simulink model "TST_ExtDem_SelectParameter"  (R2016b)
settings: Solver=FixedStepDiscrete  StartTime=0.0  StopTime=simTime  FixedStep=sampleTime  RelTol=1e-3
values from neighbouring files (symbols this model uses):
  testCase = 1    [initTST_ExtDem_SelectParameter_001.m]
libraries: simulink x34, UnitTest_Lib x32
(part 1 of 2)
settings Model: Creator=dulinggang  LastModifiedBy=dulinggang
settings DebuggingCC: SignalRangeChecking=error

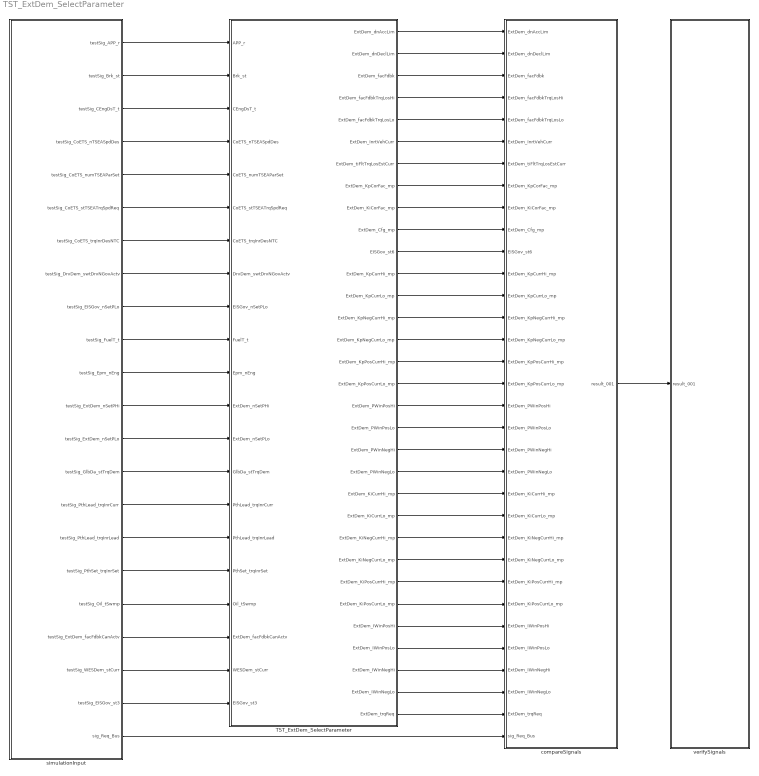
== system TST_ExtDem_SelectParameter ==
  TST_ExtDem_SelectParameter : Subsystem
  compareSignals : Subsystem
  simulationInput : Subsystem
  verifySignals : Subsystem
  wires:
  simulationInput/1(testSig_APP_r) -> TST_ExtDem_SelectParameter/1(APP_r)
  simulationInput/2(testSig_Brk_st) -> TST_ExtDem_SelectParameter/2(Brk_st)
  simulationInput/3(testSig_CEngDsT_t) -> TST_ExtDem_SelectParameter/3(CEngDsT_t)
  simulationInput/4(testSig_CoETS_nTSEASpdDes) -> TST_ExtDem_SelectParameter/4(CoETS_nTSEASpdDes)
  simulationInput/5(testSig_CoETS_numTSEAParSet) -> TST_ExtDem_SelectParameter/5(CoETS_numTSEAParSet)
  simulationInput/6(testSig_CoETS_stTSEATrqSpdReq) -> TST_ExtDem_SelectParameter/6(CoETS_stTSEATrqSpdReq)
  simulationInput/7(testSig_CoETS_trqInrDesNTC) -> TST_ExtDem_SelectParameter/7(CoETS_trqInrDesNTC)
  simulationInput/8(testSig_DrvDem_swtDrvNGovActv) -> TST_ExtDem_SelectParameter/8(DrvDem_swtDrvNGovActv)
  simulationInput/9(testSig_EISGov_nSetPLo) -> TST_ExtDem_SelectParameter/9(EISGov_nSetPLo)
  simulationInput/10(testSig_FuelT_t) -> TST_ExtDem_SelectParameter/10(FuelT_t)
  simulationInput/11(testSig_Epm_nEng) -> TST_ExtDem_SelectParameter/11(Epm_nEng)
  simulationInput/12(testSig_ExtDem_nSetPHi) -> TST_ExtDem_SelectParameter/12(ExtDem_nSetPHi)
  simulationInput/13(testSig_ExtDem_nSetPLo) -> TST_ExtDem_SelectParameter/13(ExtDem_nSetPLo)
  simulationInput/14(testSig_GlbDa_stTrqDem) -> TST_ExtDem_SelectParameter/14(GlbDa_stTrqDem)
  simulationInput/15(testSig_PthLead_trqInrCurr) -> TST_ExtDem_SelectParameter/15(PthLead_trqInrCurr)
  simulationInput/16(testSig_PthLead_trqInrLead) -> TST_ExtDem_SelectParameter/16(PthLead_trqInrLead)
  simulationInput/17(testSig_PthSet_trqInrSet) -> TST_ExtDem_SelectParameter/17(PthSet_trqInrSet)
  simulationInput/18(testSig_Oil_tSwmp) -> TST_ExtDem_SelectParameter/18(Oil_tSwmp)
  simulationInput/19(testSig_ExtDem_facFdbkCanActv) -> TST_ExtDem_SelectParameter/19(ExtDem_facFdbkCanActv)
  simulationInput/20(testSig_WESDem_stCurr) -> TST_ExtDem_SelectParameter/20(WESDem_stCurr)
  simulationInput/21(testSig_EISGov_st3) -> TST_ExtDem_SelectParameter/21(EISGov_st3)
  TST_ExtDem_SelectParameter/1(ExtDem_dnAccLim) -> compareSignals/1(ExtDem_dnAccLim)
  TST_ExtDem_SelectParameter/2(ExtDem_dnDeclLim) -> compareSignals/2(ExtDem_dnDeclLim)
  TST_ExtDem_SelectParameter/3(ExtDem_facFdbk) -> compareSignals/3(ExtDem_facFdbk)
  TST_ExtDem_SelectParameter/4(ExtDem_facFdbkTrqLosHi) -> compareSignals/4(ExtDem_facFdbkTrqLosHi)
  TST_ExtDem_SelectParameter/5(ExtDem_facFdbkTrqLosLo) -> compareSignals/5(ExtDem_facFdbkTrqLosLo)
  TST_ExtDem_SelectParameter/6(ExtDem_InrtVehCurr) -> compareSignals/6(ExtDem_InrtVehCurr)
  TST_ExtDem_SelectParameter/7(ExtDem_tiFltTrqLosEstCurr) -> compareSignals/7(ExtDem_tiFltTrqLosEstCurr)
  TST_ExtDem_SelectParameter/8(ExtDem_KpCorFac_mp) -> compareSignals/8(ExtDem_KpCorFac_mp)
  TST_ExtDem_SelectParameter/9(ExtDem_KiCorFac_mp) -> compareSignals/9(ExtDem_KiCorFac_mp)
  TST_ExtDem_SelectParameter/10(ExtDem_Cfg_mp) -> compareSignals/10(ExtDem_Cfg_mp)
  TST_ExtDem_SelectParameter/11(EISGov_st6) -> compareSignals/11(EISGov_st6)
  TST_ExtDem_SelectParameter/12(ExtDem_KpCurrHi_mp) -> compareSignals/12(ExtDem_KpCurrHi_mp)
  TST_ExtDem_SelectParameter/13(ExtDem_KpCurrLo_mp) -> compareSignals/13(ExtDem_KpCurrLo_mp)
  TST_ExtDem_SelectParameter/14(ExtDem_KpNegCurrHi_mp) -> compareSignals/14(ExtDem_KpNegCurrHi_mp)
  TST_ExtDem_SelectParameter/15(ExtDem_KpNegCurrLo_mp) -> compareSignals/15(ExtDem_KpNegCurrLo_mp)
  TST_ExtDem_SelectParameter/16(ExtDem_KpPosCurrHi_mp) -> compareSignals/16(ExtDem_KpPosCurrHi_mp)
  TST_ExtDem_SelectParameter/17(ExtDem_KpPosCurrLo_mp) -> compareSignals/17(ExtDem_KpPosCurrLo_mp)
  TST_ExtDem_SelectParameter/18(ExtDem_PWinPosHi) -> compareSignals/18(ExtDem_PWinPosHi)
  TST_ExtDem_SelectParameter/19(ExtDem_PWinPosLo) -> compareSignals/19(ExtDem_PWinPosLo)
  TST_ExtDem_SelectParameter/20(ExtDem_PWinNegHi) -> compareSignals/20(ExtDem_PWinNegHi)
  TST_ExtDem_SelectParameter/21(ExtDem_PWinNegLo) -> compareSignals/21(ExtDem_PWinNegLo)
  TST_ExtDem_SelectParameter/22(ExtDem_KiCurrHi_mp) -> compareSignals/22(ExtDem_KiCurrHi_mp)
  TST_ExtDem_SelectParameter/23(ExtDem_KiCurrLo_mp) -> compareSignals/23(ExtDem_KiCurrLo_mp)
  TST_ExtDem_SelectParameter/24(ExtDem_KiNegCurrHi_mp) -> compareSignals/24(ExtDem_KiNegCurrHi_mp)
  TST_ExtDem_SelectParameter/25(ExtDem_KiNegCurrLo_mp) -> compareSignals/25(ExtDem_KiNegCurrLo_mp)
  TST_ExtDem_SelectParameter/26(ExtDem_KiPosCurrHi_mp) -> compareSignals/26(ExtDem_KiPosCurrHi_mp)
  TST_ExtDem_SelectParameter/27(ExtDem_KiPosCurrLo_mp) -> compareSignals/27(ExtDem_KiPosCurrLo_mp)
  TST_ExtDem_SelectParameter/28(ExtDem_IWinPosHi) -> compareSignals/28(ExtDem_IWinPosHi)
  TST_ExtDem_SelectParameter/29(ExtDem_IWinPosLo) -> compareSignals/29(ExtDem_IWinPosLo)
  TST_ExtDem_SelectParameter/30(ExtDem_IWinNegHi) -> compareSignals/30(ExtDem_IWinNegHi)
  TST_ExtDem_SelectParameter/31(ExtDem_IWinNegLo) -> compareSignals/31(ExtDem_IWinNegLo)
  TST_ExtDem_SelectParameter/32(ExtDem_trqReq) -> compareSignals/32(ExtDem_trqReq)
  simulationInput/22(sig_Req_Bus) -> compareSignals/33(sig_Req_Bus)
  compareSignals/1(result_001) -> verifySignals/1(result_001)

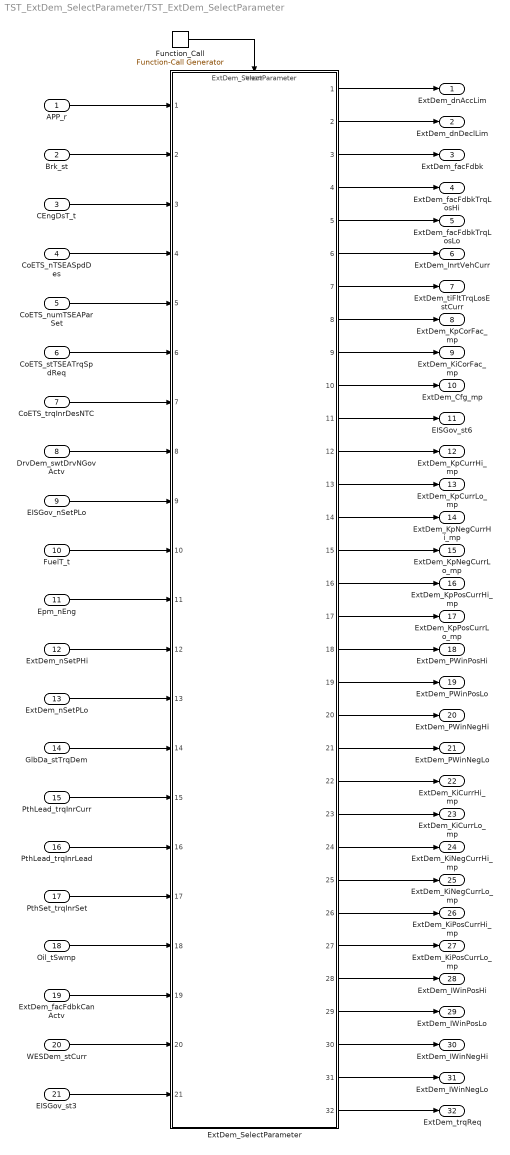
== system TST_ExtDem_SelectParameter/TST_ExtDem_SelectParameter ==
  APP_r : Inport
  Brk_st : Inport  Port=2
  CEngDsT_t : Inport  Port=3
  CoETS_nTSEASpdDes : Inport  Port=4
  CoETS_numTSEAParSet : Inport  Port=5
  CoETS_stTSEATrqSpdReq : Inport  Port=6
  CoETS_trqInrDesNTC : Inport  Port=7
  DrvDem_swtDrvNGovActv : Inport  Port=8
  EISGov_nSetPLo : Inport  Port=9
  FuelT_t : Inport  Port=10
  Epm_nEng : Inport  Port=11
  ExtDem_nSetPHi : Inport  Port=12
  ExtDem_nSetPLo : Inport  Port=13
  GlbDa_stTrqDem : Inport  Port=14
  PthLead_trqInrCurr : Inport  Port=15
  PthLead_trqInrLead : Inport  Port=16
  PthSet_trqInrSet : Inport  Port=17
  Oil_tSwmp : Inport  Port=18
  ExtDem_facFdbkCanActv : Inport  Port=19
  WESDem_stCurr : Inport  Port=20
  EISGov_st3 : Inport  Port=21
  ExtDem_SelectParameter : ModelReference  ModelNameDialog=ExtDem_SelectParameter  SimulationMode=Normal  ModelReferenceVersion=1.171  TriggerPortName=function  TriggerPortTriggerType=function-call  TriggerPortStatesWhenEnabling=held
  Function_Call : simulink/Ports & Subsystems/Function-Call Generator  sample_time=sampleTime  numberOfIterations=1
  ExtDem_dnAccLim : Outport
  ExtDem_dnDeclLim : Outport  Port=2
  ExtDem_facFdbk : Outport  Port=3
  ExtDem_facFdbkTrqLosHi : Outport  Port=4
  ExtDem_facFdbkTrqLosLo : Outport  Port=5
  ExtDem_InrtVehCurr : Outport  Port=6
  ExtDem_tiFltTrqLosEstCurr : Outport  Port=7
  ExtDem_KpCorFac_mp : Outport  Port=8
  ExtDem_KiCorFac_mp : Outport  Port=9
  ExtDem_Cfg_mp : Outport  Port=10
  EISGov_st6 : Outport  Port=11
  ExtDem_KpCurrHi_mp : Outport  Port=12
  ExtDem_KpCurrLo_mp : Outport  Port=13
  ExtDem_KpNegCurrHi_mp : Outport  Port=14
  ExtDem_KpNegCurrLo_mp : Outport  Port=15
  ExtDem_KpPosCurrHi_mp : Outport  Port=16
  ExtDem_KpPosCurrLo_mp : Outport  Port=17
  ExtDem_PWinPosHi : Outport  Port=18
  ExtDem_PWinPosLo : Outport  Port=19
  ExtDem_PWinNegHi : Outport  Port=20
  ExtDem_PWinNegLo : Outport  Port=21
  ExtDem_KiCurrHi_mp : Outport  Port=22
  ExtDem_KiCurrLo_mp : Outport  Port=23
  ExtDem_KiNegCurrHi_mp : Outport  Port=24
  ExtDem_KiNegCurrLo_mp : Outport  Port=25
  ExtDem_KiPosCurrHi_mp : Outport  Port=26
  ExtDem_KiPosCurrLo_mp : Outport  Port=27
  ExtDem_IWinPosHi : Outport  Port=28
  ExtDem_IWinPosLo : Outport  Port=29
  ExtDem_IWinNegHi : Outport  Port=30
  ExtDem_IWinNegLo : Outport  Port=31
  ExtDem_trqReq : Outport  Port=32
  wires:
  Function_Call/1 -> ExtDem_SelectParameter/Trigger
  APP_r/1 -> ExtDem_SelectParameter/1
  Brk_st/1 -> ExtDem_SelectParameter/2
  CEngDsT_t/1 -> ExtDem_SelectParameter/3
  CoETS_nTSEASpdDes/1 -> ExtDem_SelectParameter/4
  CoETS_numTSEAParSet/1 -> ExtDem_SelectParameter/5
  CoETS_stTSEATrqSpdReq/1 -> ExtDem_SelectParameter/6
  CoETS_trqInrDesNTC/1 -> ExtDem_SelectParameter/7
  DrvDem_swtDrvNGovActv/1 -> ExtDem_SelectParameter/8
  EISGov_nSetPLo/1 -> ExtDem_SelectParameter/9
  FuelT_t/1 -> ExtDem_SelectParameter/10
  Epm_nEng/1 -> ExtDem_SelectParameter/11
  ExtDem_nSetPHi/1 -> ExtDem_SelectParameter/12
  ExtDem_nSetPLo/1 -> ExtDem_SelectParameter/13
  GlbDa_stTrqDem/1 -> ExtDem_SelectParameter/14
  PthLead_trqInrCurr/1 -> ExtDem_SelectParameter/15
  PthLead_trqInrLead/1 -> ExtDem_SelectParameter/16
  PthSet_trqInrSet/1 -> ExtDem_SelectParameter/17
  Oil_tSwmp/1 -> ExtDem_SelectParameter/18
  ExtDem_facFdbkCanActv/1 -> ExtDem_SelectParameter/19
  WESDem_stCurr/1 -> ExtDem_SelectParameter/20
  EISGov_st3/1 -> ExtDem_SelectParameter/21
  ExtDem_SelectParameter/1 -> ExtDem_dnAccLim/1
  ExtDem_SelectParameter/2 -> ExtDem_dnDeclLim/1
  ExtDem_SelectParameter/3 -> ExtDem_facFdbk/1
  ExtDem_SelectParameter/4 -> ExtDem_facFdbkTrqLosHi/1
  ExtDem_SelectParameter/5 -> ExtDem_facFdbkTrqLosLo/1
  ExtDem_SelectParameter/6 -> ExtDem_InrtVehCurr/1
  ExtDem_SelectParameter/7 -> ExtDem_tiFltTrqLosEstCurr/1
  ExtDem_SelectParameter/8 -> ExtDem_KpCorFac_mp/1
  ExtDem_SelectParameter/9 -> ExtDem_KiCorFac_mp/1
  ExtDem_SelectParameter/10 -> ExtDem_Cfg_mp/1
  ExtDem_SelectParameter/11 -> EISGov_st6/1
  ExtDem_SelectParameter/12 -> ExtDem_KpCurrHi_mp/1
  ExtDem_SelectParameter/13 -> ExtDem_KpCurrLo_mp/1
  ExtDem_SelectParameter/14 -> ExtDem_KpNegCurrHi_mp/1
  ExtDem_SelectParameter/15 -> ExtDem_KpNegCurrLo_mp/1
  ExtDem_SelectParameter/16 -> ExtDem_KpPosCurrHi_mp/1
  ExtDem_SelectParameter/17 -> ExtDem_KpPosCurrLo_mp/1
  ExtDem_SelectParameter/18 -> ExtDem_PWinPosHi/1
  ExtDem_SelectParameter/19 -> ExtDem_PWinPosLo/1
  ExtDem_SelectParameter/20 -> ExtDem_PWinNegHi/1
  ExtDem_SelectParameter/21 -> ExtDem_PWinNegLo/1
  ExtDem_SelectParameter/22 -> ExtDem_KiCurrHi_mp/1
  ExtDem_SelectParameter/23 -> ExtDem_KiCurrLo_mp/1
  ExtDem_SelectParameter/24 -> ExtDem_KiNegCurrHi_mp/1
  ExtDem_SelectParameter/25 -> ExtDem_KiNegCurrLo_mp/1
  ExtDem_SelectParameter/26 -> ExtDem_KiPosCurrHi_mp/1
  ExtDem_SelectParameter/27 -> ExtDem_KiPosCurrLo_mp/1
  ExtDem_SelectParameter/28 -> ExtDem_IWinPosHi/1
  ExtDem_SelectParameter/29 -> ExtDem_IWinPosLo/1
  ExtDem_SelectParameter/30 -> ExtDem_IWinNegHi/1
  ExtDem_SelectParameter/31 -> ExtDem_IWinNegLo/1
  ExtDem_SelectParameter/32 -> ExtDem_trqReq/1

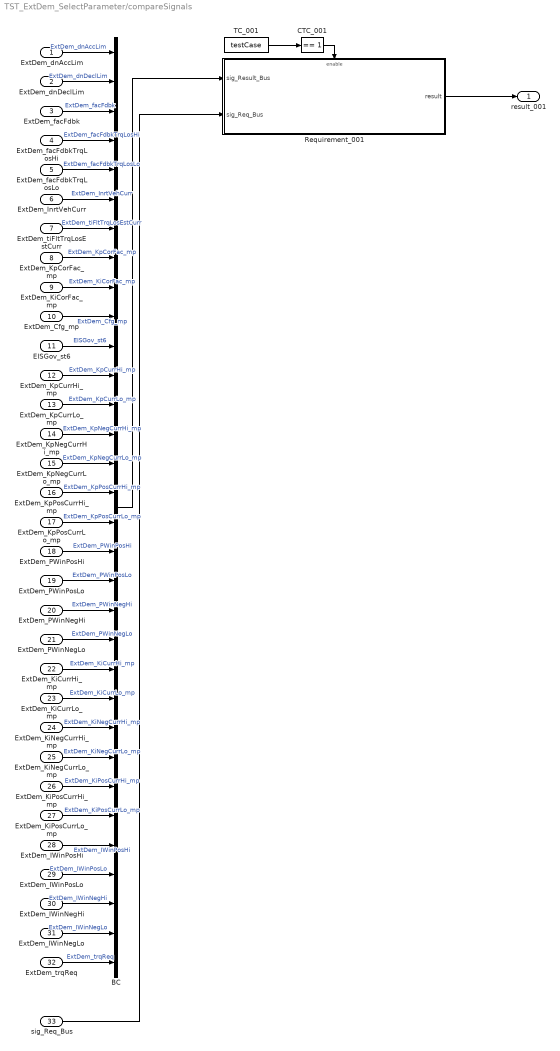
== system TST_ExtDem_SelectParameter/compareSignals ==
  ExtDem_dnAccLim : Inport
  ExtDem_dnDeclLim : Inport  Port=2
  ExtDem_facFdbk : Inport  Port=3
  ExtDem_facFdbkTrqLosHi : Inport  Port=4
  ExtDem_facFdbkTrqLosLo : Inport  Port=5
  ExtDem_InrtVehCurr : Inport  Port=6
  ExtDem_tiFltTrqLosEstCurr : Inport  Port=7
  ExtDem_KpCorFac_mp : Inport  Port=8
  ExtDem_KiCorFac_mp : Inport  Port=9
  ExtDem_Cfg_mp : Inport  Port=10
  EISGov_st6 : Inport  Port=11
  ExtDem_KpCurrHi_mp : Inport  Port=12
  ExtDem_KpCurrLo_mp : Inport  Port=13
  ExtDem_KpNegCurrHi_mp : Inport  Port=14
  ExtDem_KpNegCurrLo_mp : Inport  Port=15
  ExtDem_KpPosCurrHi_mp : Inport  Port=16
  ExtDem_KpPosCurrLo_mp : Inport  Port=17
  ExtDem_PWinPosHi : Inport  Port=18
  ExtDem_PWinPosLo : Inport  Port=19
  ExtDem_PWinNegHi : Inport  Port=20
  ExtDem_PWinNegLo : Inport  Port=21
  ExtDem_KiCurrHi_mp : Inport  Port=22
  ExtDem_KiCurrLo_mp : Inport  Port=23
  ExtDem_KiNegCurrHi_mp : Inport  Port=24
  ExtDem_KiNegCurrLo_mp : Inport  Port=25
  ExtDem_KiPosCurrHi_mp : Inport  Port=26
  ExtDem_KiPosCurrLo_mp : Inport  Port=27
  ExtDem_IWinPosHi : Inport  Port=28
  ExtDem_IWinPosLo : Inport  Port=29
  ExtDem_IWinNegHi : Inport  Port=30
  ExtDem_IWinNegLo : Inport  Port=31
  ExtDem_trqReq : Inport  Port=32
  sig_Req_Bus : Inport  Port=33
  BC : BusCreator  Inputs=32
  CTC_001 : simulink/Logic and Bit Operations/Compare To Constant  relop===  const=1  OutDataTypeStr=boolean
  Requirement_001 : Subsystem
  TC_001 : Constant  Value=testCase
  result_001 : Outport
  wires:
  ExtDem_dnAccLim/1 -> BC/1  "ExtDem_dnAccLim"
  ExtDem_dnDeclLim/1 -> BC/2  "ExtDem_dnDeclLim"
  ExtDem_facFdbk/1 -> BC/3  "ExtDem_facFdbk"
  ExtDem_facFdbkTrqLosHi/1 -> BC/4  "ExtDem_facFdbkTrqLosHi"
  ExtDem_facFdbkTrqLosLo/1 -> BC/5  "ExtDem_facFdbkTrqLosLo"
  ExtDem_InrtVehCurr/1 -> BC/6  "ExtDem_InrtVehCurr"
  ExtDem_tiFltTrqLosEstCurr/1 -> BC/7  "ExtDem_tiFltTrqLosEstCurr"
  ExtDem_KpCorFac_mp/1 -> BC/8  "ExtDem_KpCorFac_mp"
  ExtDem_KiCorFac_mp/1 -> BC/9  "ExtDem_KiCorFac_mp"
  ExtDem_Cfg_mp/1 -> BC/10  "ExtDem_Cfg_mp"
  EISGov_st6/1 -> BC/11  "EISGov_st6"
  ExtDem_KpCurrHi_mp/1 -> BC/12  "ExtDem_KpCurrHi_mp"
  ExtDem_KpCurrLo_mp/1 -> BC/13  "ExtDem_KpCurrLo_mp"
  ExtDem_KpNegCurrHi_mp/1 -> BC/14  "ExtDem_KpNegCurrHi_mp"
  ExtDem_KpNegCurrLo_mp/1 -> BC/15  "ExtDem_KpNegCurrLo_mp"
  ExtDem_KpPosCurrHi_mp/1 -> BC/16  "ExtDem_KpPosCurrHi_mp"
  ExtDem_KpPosCurrLo_mp/1 -> BC/17  "ExtDem_KpPosCurrLo_mp"
  ExtDem_PWinPosHi/1 -> BC/18  "ExtDem_PWinPosHi"
  ExtDem_PWinPosLo/1 -> BC/19  "ExtDem_PWinPosLo"
  ExtDem_PWinNegHi/1 -> BC/20  "ExtDem_PWinNegHi"
  ExtDem_PWinNegLo/1 -> BC/21  "ExtDem_PWinNegLo"
  ExtDem_KiCurrHi_mp/1 -> BC/22  "ExtDem_KiCurrHi_mp"
  ExtDem_KiCurrLo_mp/1 -> BC/23  "ExtDem_KiCurrLo_mp"
  ExtDem_KiNegCurrHi_mp/1 -> BC/24  "ExtDem_KiNegCurrHi_mp"
  ExtDem_KiNegCurrLo_mp/1 -> BC/25  "ExtDem_KiNegCurrLo_mp"
  ExtDem_KiPosCurrHi_mp/1 -> BC/26  "ExtDem_KiPosCurrHi_mp"
  ExtDem_KiPosCurrLo_mp/1 -> BC/27  "ExtDem_KiPosCurrLo_mp"
  ExtDem_IWinPosHi/1 -> BC/28  "ExtDem_IWinPosHi"
  ExtDem_IWinPosLo/1 -> BC/29  "ExtDem_IWinPosLo"
  ExtDem_IWinNegHi/1 -> BC/30  "ExtDem_IWinNegHi"
  ExtDem_IWinNegLo/1 -> BC/31  "ExtDem_IWinNegLo"
  ExtDem_trqReq/1 -> BC/32  "ExtDem_trqReq"
  TC_001/1 -> CTC_001/1
  CTC_001/1 -> Requirement_001/Enable
  sig_Req_Bus/1 -> Requirement_001/2(sig_Req_Bus)
  BC/1 -> Requirement_001/1(sig_Result_Bus)
  Requirement_001/1(result) -> result_001/1

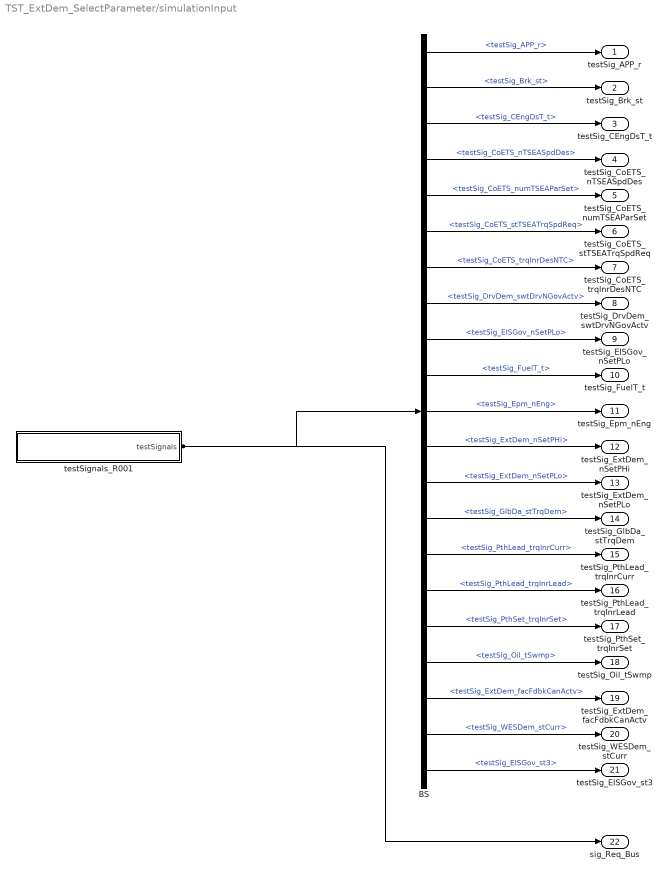
== system TST_ExtDem_SelectParameter/simulationInput ==
  BS : BusSelector  OutputSignals=testSig_APP_r,testSig_Brk_st,testSig_CEngDsT_t,testSig_CoETS_nTSEASpdDes,testSig_CoETS_numTSEAParSet,testSig_CoETS_stTSEATrqSpdReq,testSig_CoETS_trqInrDesNTC,testSig_DrvDem_swtDrvNGovActv,testSig_EISGov_nSetPLo,testSig_FuelT_t,testSig_Epm_nEng,testSig_ExtDem_nSetPHi,testSig_ExtDem_nSetPLo,testSig_GlbDa_stTrqDem,testSig_PthLead_trqInrCurr,testSig_PthLead_trqInrLead,testSig_PthSet_trqInrSet,testSig_Oil_tSwmp,testSig_ExtDem_facFdbkCanActv,testSig_WESDem_stCurr,testSig_EISGov_st3
  testSignals_R001 : Subsystem
  testSig_APP_r : Outport
  testSig_Brk_st : Outport  Port=2
  testSig_CEngDsT_t : Outport  Port=3
  testSig_CoETS_nTSEASpdDes : Outport  Port=4
  testSig_CoETS_numTSEAParSet : Outport  Port=5
  testSig_CoETS_stTSEATrqSpdReq : Outport  Port=6
  testSig_CoETS_trqInrDesNTC : Outport  Port=7
  testSig_DrvDem_swtDrvNGovActv : Outport  Port=8
  testSig_EISGov_nSetPLo : Outport  Port=9
  testSig_FuelT_t : Outport  Port=10
  testSig_Epm_nEng : Outport  Port=11
  testSig_ExtDem_nSetPHi : Outport  Port=12
  testSig_ExtDem_nSetPLo : Outport  Port=13
  testSig_GlbDa_stTrqDem : Outport  Port=14
  testSig_PthLead_trqInrCurr : Outport  Port=15
  testSig_PthLead_trqInrLead : Outport  Port=16
  testSig_PthSet_trqInrSet : Outport  Port=17
  testSig_Oil_tSwmp : Outport  Port=18
  testSig_ExtDem_facFdbkCanActv : Outport  Port=19
  testSig_WESDem_stCurr : Outport  Port=20
  testSig_EISGov_st3 : Outport  Port=21
  sig_Req_Bus : Outport  Port=22
  wires:
  BS/1 -> testSig_APP_r/1  "<testSig_APP_r>"
  BS/2 -> testSig_Brk_st/1  "<testSig_Brk_st>"
  BS/3 -> testSig_CEngDsT_t/1  "<testSig_CEngDsT_t>"
  BS/4 -> testSig_CoETS_nTSEASpdDes/1  "<testSig_CoETS_nTSEASpdDes>"
  BS/5 -> testSig_CoETS_numTSEAParSet/1  "<testSig_CoETS_numTSEAParSet>"
  BS/6 -> testSig_CoETS_stTSEATrqSpdReq/1  "<testSig_CoETS_stTSEATrqSpdReq>"
  BS/7 -> testSig_CoETS_trqInrDesNTC/1  "<testSig_CoETS_trqInrDesNTC>"
  BS/8 -> testSig_DrvDem_swtDrvNGovActv/1  "<testSig_DrvDem_swtDrvNGovActv>"
  BS/9 -> testSig_EISGov_nSetPLo/1  "<testSig_EISGov_nSetPLo>"
  BS/10 -> testSig_FuelT_t/1  "<testSig_FuelT_t>"
  BS/11 -> testSig_Epm_nEng/1  "<testSig_Epm_nEng>"
  BS/12 -> testSig_ExtDem_nSetPHi/1  "<testSig_ExtDem_nSetPHi>"
  BS/13 -> testSig_ExtDem_nSetPLo/1  "<testSig_ExtDem_nSetPLo>"
  BS/14 -> testSig_GlbDa_stTrqDem/1  "<testSig_GlbDa_stTrqDem>"
  BS/15 -> testSig_PthLead_trqInrCurr/1  "<testSig_PthLead_trqInrCurr>"
  BS/16 -> testSig_PthLead_trqInrLead/1  "<testSig_PthLead_trqInrLead>"
  BS/17 -> testSig_PthSet_trqInrSet/1  "<testSig_PthSet_trqInrSet>"
  BS/18 -> testSig_Oil_tSwmp/1  "<testSig_Oil_tSwmp>"
  BS/19 -> testSig_ExtDem_facFdbkCanActv/1  "<testSig_ExtDem_facFdbkCanActv>"
  BS/20 -> testSig_WESDem_stCurr/1  "<testSig_WESDem_stCurr>"
  BS/21 -> testSig_EISGov_st3/1  "<testSig_EISGov_st3>"
  testSignals_R001/1(testSignals) -> BS/1, sig_Req_Bus/1

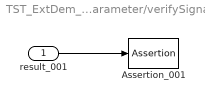
== system TST_ExtDem_SelectParameter/verifySignals ==
  result_001 : Inport
  Assertion_001 : Assertion  Enabled=off
  wires:
  result_001/1 -> Assertion_001/1

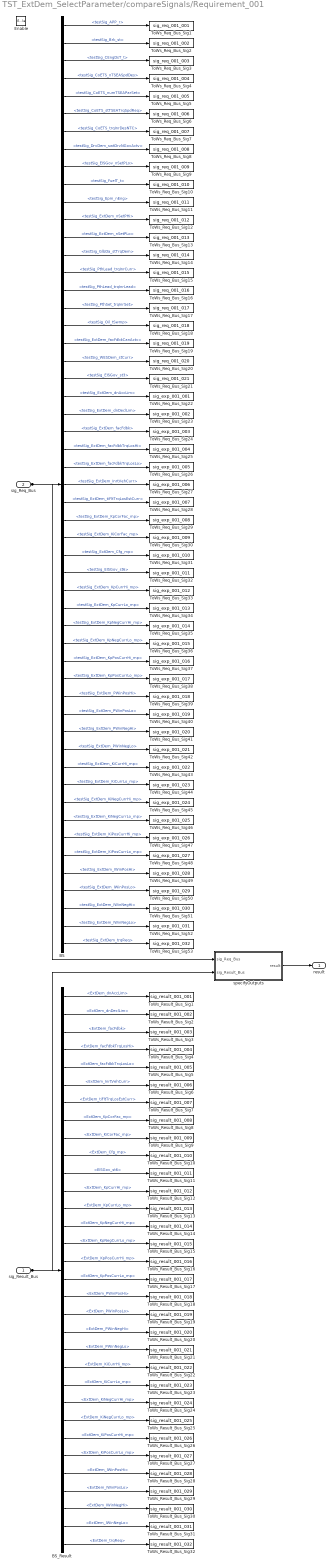
== system TST_ExtDem_SelectParameter/compareSignals/Requirement_001 ==
  sig_Result_Bus : Inport
  sig_Req_Bus : Inport  Port=2
  Enable : EnablePort
  BS : BusSelector  OutputSignals=testSig_APP_r,testSig_Brk_st,testSig_CEngDsT_t,testSig_CoETS_nTSEASpdDes,testSig_CoETS_numTSEAParSet,testSig_CoETS_stTSEATrqSpdReq,testSig_CoETS_trqInrDesNTC,testSig_DrvDem_swtDrvNGovActv,testSig_EISGov_nSetPLo,testSig_FuelT_t,testSig_Epm_nEng,testSig_ExtDem_nSetPHi,testSig_ExtDem_nSetPLo,testSig_GlbDa_stTrqDem,testSig_PthLead_trqInrCurr,testSig_PthLead_trqInrLead,testSig_PthSet_trqInrSet,testSig_Oil_tSwmp,testSig_ExtDem_facFdbkCanActv,testSig_WESDem_stCurr,testSig_EISGov_st3,testSig_ExtDem_dnAccLim,testSig_ExtDem_dnDeclLim,testSig_ExtDem_facFdbk,testSig_ExtDem_facFdbkTrqLosHi,testSig_ExtDem_facFdbkTrqLosLo,testSig_ExtDem_InrtVehCurr,testSig_ExtDem_tiFltTrqLosEstCurr,testSig_ExtDem_KpCorFac_mp,testSig_ExtDem_KiCorFac_mp,testSig_ExtDem_Cfg_mp,testSig_EISGov_st6,testSig_ExtDem_KpCurrHi_mp,testSig_ExtDem_KpCurrLo_mp,testSig_ExtDem_KpNegCurrHi_mp,testSig_ExtDem_KpNegCurrLo_mp,testSig_ExtDem_KpPosCurrHi_mp,testSig_ExtDem_KpPosCurrLo_mp,testSig_ExtDem_PWinPosHi,testSig_ExtDem_PWinPosLo,testSig_ExtDem_PWinNegHi,testSig_ExtDem_PWinNegLo,testSig_ExtDem_KiCurrHi_mp,testSig_ExtDem_KiCurrLo_mp,testSig_ExtDem_KiNegCurrHi_mp,testSig_ExtDem_KiNegCurrLo_mp,testSig_ExtDem_KiPosCurrHi_mp,testSig_ExtDem_KiPosCurrLo_mp,testSig_ExtDem_IWinPosHi,testSig_ExtDem_IWinPosLo,testSig_ExtDem_IWinNegHi,testSig_ExtDem_IWinNegLo,testSig_ExtDem_trqReq
  BS_Result : BusSelector  OutputSignals=ExtDem_dnAccLim,ExtDem_dnDeclLim,ExtDem_facFdbk,ExtDem_facFdbkTrqLosHi,ExtDem_facFdbkTrqLosLo,ExtDem_InrtVehCurr,ExtDem_tiFltTrqLosEstCurr,ExtDem_KpCorFac_mp,ExtDem_KiCorFac_mp,ExtDem_Cfg_mp,EISGov_st6,ExtDem_KpCurrHi_mp,ExtDem_KpCurrLo_mp,ExtDem_KpNegCurrHi_mp,ExtDem_KpNegCurrLo_mp,ExtDem_KpPosCurrHi_mp,ExtDem_KpPosCurrLo_mp,ExtDem_PWinPosHi,ExtDem_PWinPosLo,ExtDem_PWinNegHi,ExtDem_PWinNegLo,ExtDem_KiCurrHi_mp,ExtDem_KiCurrLo_mp,ExtDem_KiNegCurrHi_mp,ExtDem_KiNegCurrLo_mp,ExtDem_KiPosCurrHi_mp,ExtDem_KiPosCurrLo_mp,ExtDem_IWinPosHi,ExtDem_IWinPosLo,ExtDem_IWinNegHi,ExtDem_IWinNegLo,ExtDem_trqReq
  ToWs_Req_Bus_Sig1 : ToWorkspace  VariableName=sig_req_001_001  SaveFormat=Structure With Time
  ToWs_Req_Bus_Sig10 : ToWorkspace  VariableName=sig_req_001_010  SaveFormat=Structure With Time
  ToWs_Req_Bus_Sig11 : ToWorkspace  VariableName=sig_req_001_011  SaveFormat=Structure With Time
  ToWs_Req_Bus_Sig12 : ToWorkspace  VariableName=sig_req_001_012  SaveFormat=Structure With Time
  ToWs_Req_Bus_Sig13 : ToWorkspace  VariableName=sig_req_001_013  SaveFormat=Structure With Time
  ToWs_Req_Bus_Sig14 : ToWorkspace  VariableName=sig_req_001_014  SaveFormat=Structure With Time
  ToWs_Req_Bus_Sig15 : ToWorkspace  VariableName=sig_req_001_015  SaveFormat=Structure With Time
  ToWs_Req_Bus_Sig16 : ToWorkspace  VariableName=sig_req_001_016  SaveFormat=Structure With Time
  ToWs_Req_Bus_Sig17 : ToWorkspace  VariableName=sig_req_001_017  SaveFormat=Structure With Time
  ToWs_Req_Bus_Sig18 : ToWorkspace  VariableName=sig_req_001_018  SaveFormat=Structure With Time
  ToWs_Req_Bus_Sig19 : ToWorkspace  VariableName=sig_req_001_019  SaveFormat=Structure With Time
  ToWs_Req_Bus_Sig2 : ToWorkspace  VariableName=sig_req_001_002  SaveFormat=Structure With Time
  ToWs_Req_Bus_Sig20 : ToWorkspace  VariableName=sig_req_001_020  SaveFormat=Structure With Time
  ToWs_Req_Bus_Sig21 : ToWorkspace  VariableName=sig_req_001_021  SaveFormat=Structure With Time
  ToWs_Req_Bus_Sig22 : ToWorkspace  VariableName=sig_exp_001_001  SaveFormat=Structure With Time
  ToWs_Req_Bus_Sig23 : ToWorkspace  VariableName=sig_exp_001_002  SaveFormat=Structure With Time
  ToWs_Req_Bus_Sig24 : ToWorkspace  VariableName=sig_exp_001_003  SaveFormat=Structure With Time
  ToWs_Req_Bus_Sig25 : ToWorkspace  VariableName=sig_exp_001_004  SaveFormat=Structure With Time
  ToWs_Req_Bus_Sig26 : ToWorkspace  VariableName=sig_exp_001_005  SaveFormat=Structure With Time
  ToWs_Req_Bus_Sig27 : ToWorkspace  VariableName=sig_exp_001_006  SaveFormat=Structure With Time
  ToWs_Req_Bus_Sig28 : ToWorkspace  VariableName=sig_exp_001_007  SaveFormat=Structure With Time
  ToWs_Req_Bus_Sig29 : ToWorkspace  VariableName=sig_exp_001_008  SaveFormat=Structure With Time
  ToWs_Req_Bus_Sig3 : ToWorkspace  VariableName=sig_req_001_003  SaveFormat=Structure With Time
  ToWs_Req_Bus_Sig30 : ToWorkspace  VariableName=sig_exp_001_009  SaveFormat=Structure With Time
  ToWs_Req_Bus_Sig31 : ToWorkspace  VariableName=sig_exp_001_010  SaveFormat=Structure With Time
  ToWs_Req_Bus_Sig32 : ToWorkspace  VariableName=sig_exp_001_011  SaveFormat=Structure With Time
  ToWs_Req_Bus_Sig33 : ToWorkspace  VariableName=sig_exp_001_012  SaveFormat=Structure With Time
  ToWs_Req_Bus_Sig34 : ToWorkspace  VariableName=sig_exp_001_013  SaveFormat=Structure With Time
  ToWs_Req_Bus_Sig35 : ToWorkspace  VariableName=sig_exp_001_014  SaveFormat=Structure With Time
  ToWs_Req_Bus_Sig36 : ToWorkspace  VariableName=sig_exp_001_015  SaveFormat=Structure With Time
  ToWs_Req_Bus_Sig37 : ToWorkspace  VariableName=sig_exp_001_016  SaveFormat=Structure With Time
  ToWs_Req_Bus_Sig38 : ToWorkspace  VariableName=sig_exp_001_017  SaveFormat=Structure With Time
  ToWs_Req_Bus_Sig39 : ToWorkspace  VariableName=sig_exp_001_018  SaveFormat=Structure With Time
  ToWs_Req_Bus_Sig4 : ToWorkspace  VariableName=sig_req_001_004  SaveFormat=Structure With Time
  ToWs_Req_Bus_Sig40 : ToWorkspace  VariableName=sig_exp_001_019  SaveFormat=Structure With Time
  ToWs_Req_Bus_Sig41 : ToWorkspace  VariableName=sig_exp_001_020  SaveFormat=Structure With Time
  ToWs_Req_Bus_Sig42 : ToWorkspace  VariableName=sig_exp_001_021  SaveFormat=Structure With Time
  ToWs_Req_Bus_Sig43 : ToWorkspace  VariableName=sig_exp_001_022  SaveFormat=Structure With Time
  ToWs_Req_Bus_Sig44 : ToWorkspace  VariableName=sig_exp_001_023  SaveFormat=Structure With Time
  ToWs_Req_Bus_Sig45 : ToWorkspace  VariableName=sig_exp_001_024  SaveFormat=Structure With Time
  ToWs_Req_Bus_Sig46 : ToWorkspace  VariableName=sig_exp_001_025  SaveFormat=Structure With Time
  ToWs_Req_Bus_Sig47 : ToWorkspace  VariableName=sig_exp_001_026  SaveFormat=Structure With Time
  ToWs_Req_Bus_Sig48 : ToWorkspace  VariableName=sig_exp_001_027  SaveFormat=Structure With Time
  ToWs_Req_Bus_Sig49 : ToWorkspace  VariableName=sig_exp_001_028  SaveFormat=Structure With Time
  ToWs_Req_Bus_Sig5 : ToWorkspace  VariableName=sig_req_001_005  SaveFormat=Structure With Time
  ToWs_Req_Bus_Sig50 : ToWorkspace  VariableName=sig_exp_001_029  SaveFormat=Structure With Time
  ToWs_Req_Bus_Sig51 : ToWorkspace  VariableName=sig_exp_001_030  SaveFormat=Structure With Time
  ToWs_Req_Bus_Sig52 : ToWorkspace  VariableName=sig_exp_001_031  SaveFormat=Structure With Time
  ToWs_Req_Bus_Sig53 : ToWorkspace  VariableName=sig_exp_001_032  SaveFormat=Structure With Time
  ToWs_Req_Bus_Sig6 : ToWorkspace  VariableName=sig_req_001_006  SaveFormat=Structure With Time
  ToWs_Req_Bus_Sig7 : ToWorkspace  VariableName=sig_req_001_007  SaveFormat=Structure With Time
  ToWs_Req_Bus_Sig8 : ToWorkspace  VariableName=sig_req_001_008  SaveFormat=Structure With Time
  ToWs_Req_Bus_Sig9 : ToWorkspace  VariableName=sig_req_001_009  SaveFormat=Structure With Time
  ToWs_Result_Bus_Sig1 : ToWorkspace  VariableName=sig_result_001_001  SaveFormat=Structure With Time
  ToWs_Result_Bus_Sig10 : ToWorkspace  VariableName=sig_result_001_010  SaveFormat=Structure With Time
  ToWs_Result_Bus_Sig11 : ToWorkspace  VariableName=sig_result_001_011  SaveFormat=Structure With Time
  ToWs_Result_Bus_Sig12 : ToWorkspace  VariableName=sig_result_001_012  SaveFormat=Structure With Time
  ToWs_Result_Bus_Sig13 : ToWorkspace  VariableName=sig_result_001_013  SaveFormat=Structure With Time
  ToWs_Result_Bus_Sig14 : ToWorkspace  VariableName=sig_result_001_014  SaveFormat=Structure With Time
  ToWs_Result_Bus_Sig15 : ToWorkspace  VariableName=sig_result_001_015  SaveFormat=Structure With Time
  ToWs_Result_Bus_Sig16 : ToWorkspace  VariableName=sig_result_001_016  SaveFormat=Structure With Time
  ToWs_Result_Bus_Sig17 : ToWorkspace  VariableName=sig_result_001_017  SaveFormat=Structure With Time
  ToWs_Result_Bus_Sig18 : ToWorkspace  VariableName=sig_result_001_018  SaveFormat=Structure With Time
  ToWs_Result_Bus_Sig19 : ToWorkspace  VariableName=sig_result_001_019  SaveFormat=Structure With Time
  ToWs_Result_Bus_Sig2 : ToWorkspace  VariableName=sig_result_001_002  SaveFormat=Structure With Time
  ToWs_Result_Bus_Sig20 : ToWorkspace  VariableName=sig_result_001_020  SaveFormat=Structure With Time
  ToWs_Result_Bus_Sig21 : ToWorkspace  VariableName=sig_result_001_021  SaveFormat=Structure With Time
  ToWs_Result_Bus_Sig22 : ToWorkspace  VariableName=sig_result_001_022  SaveFormat=Structure With Time
  ToWs_Result_Bus_Sig23 : ToWorkspace  VariableName=sig_result_001_023  SaveFormat=Structure With Time
  ToWs_Result_Bus_Sig24 : ToWorkspace  VariableName=sig_result_001_024  SaveFormat=Structure With Time
  ToWs_Result_Bus_Sig25 : ToWorkspace  VariableName=sig_result_001_025  SaveFormat=Structure With Time
  ToWs_Result_Bus_Sig26 : ToWorkspace  VariableName=sig_result_001_026  SaveFormat=Structure With Time
  ToWs_Result_Bus_Sig27 : ToWorkspace  VariableName=sig_result_001_027  SaveFormat=Structure With Time
  ToWs_Result_Bus_Sig28 : ToWorkspace  VariableName=sig_result_001_028  SaveFormat=Structure With Time
  ToWs_Result_Bus_Sig29 : ToWorkspace  VariableName=sig_result_001_029  SaveFormat=Structure With Time
  ToWs_Result_Bus_Sig3 : ToWorkspace  VariableName=sig_result_001_003  SaveFormat=Structure With Time
  ToWs_Result_Bus_Sig30 : ToWorkspace  VariableName=sig_result_001_030  SaveFormat=Structure With Time
  ToWs_Result_Bus_Sig31 : ToWorkspace  VariableName=sig_result_001_031  SaveFormat=Structure With Time
  ToWs_Result_Bus_Sig32 : ToWorkspace  VariableName=sig_result_001_032  SaveFormat=Structure With Time
  ToWs_Result_Bus_Sig4 : ToWorkspace  VariableName=sig_result_001_004  SaveFormat=Structure With Time
  ToWs_Result_Bus_Sig5 : ToWorkspace  VariableName=sig_result_001_005  SaveFormat=Structure With Time
  ToWs_Result_Bus_Sig6 : ToWorkspace  VariableName=sig_result_001_006  SaveFormat=Structure With Time
  ToWs_Result_Bus_Sig7 : ToWorkspace  VariableName=sig_result_001_007  SaveFormat=Structure With Time
  ToWs_Result_Bus_Sig8 : ToWorkspace  VariableName=sig_result_001_008  SaveFormat=Structure With Time
  ToWs_Result_Bus_Sig9 : ToWorkspace  VariableName=sig_result_001_009  SaveFormat=Structure With Time
  specifyOutputs : Subsystem
  result : Outport
  wires:
  sig_Req_Bus/1 -> BS/1, specifyOutputs/1(sig_Req_Bus)
  BS/1 -> ToWs_Req_Bus_Sig1/1  "<testSig_APP_r>"
  BS/2 -> ToWs_Req_Bus_Sig2/1  "<testSig_Brk_st>"
  BS/3 -> ToWs_Req_Bus_Sig3/1  "<testSig_CEngDsT_t>"
  BS/4 -> ToWs_Req_Bus_Sig4/1  "<testSig_CoETS_nTSEASpdDes>"
  BS/5 -> ToWs_Req_Bus_Sig5/1  "<testSig_CoETS_numTSEAParSet>"
  BS/6 -> ToWs_Req_Bus_Sig6/1  "<testSig_CoETS_stTSEATrqSpdReq>"
  BS/7 -> ToWs_Req_Bus_Sig7/1  "<testSig_CoETS_trqInrDesNTC>"
  BS/8 -> ToWs_Req_Bus_Sig8/1  "<testSig_DrvDem_swtDrvNGovActv>"
  BS/9 -> ToWs_Req_Bus_Sig9/1  "<testSig_EISGov_nSetPLo>"
  BS/10 -> ToWs_Req_Bus_Sig10/1  "<testSig_FuelT_t>"
  BS/11 -> ToWs_Req_Bus_Sig11/1  "<testSig_Epm_nEng>"
  BS/12 -> ToWs_Req_Bus_Sig12/1  "<testSig_ExtDem_nSetPHi>"
  BS/13 -> ToWs_Req_Bus_Sig13/1  "<testSig_ExtDem_nSetPLo>"
  BS/14 -> ToWs_Req_Bus_Sig14/1  "<testSig_GlbDa_stTrqDem>"
  BS/15 -> ToWs_Req_Bus_Sig15/1  "<testSig_PthLead_trqInrCurr>"
  BS/16 -> ToWs_Req_Bus_Sig16/1  "<testSig_PthLead_trqInrLead>"
  BS/17 -> ToWs_Req_Bus_Sig17/1  "<testSig_PthSet_trqInrSet>"
  BS/18 -> ToWs_Req_Bus_Sig18/1  "<testSig_Oil_tSwmp>"
  BS/19 -> ToWs_Req_Bus_Sig19/1  "<testSig_ExtDem_facFdbkCanActv>"
  BS/20 -> ToWs_Req_Bus_Sig20/1  "<testSig_WESDem_stCurr>"
  BS/21 -> ToWs_Req_Bus_Sig21/1  "<testSig_EISGov_st3>"
  BS/22 -> ToWs_Req_Bus_Sig22/1  "<testSig_ExtDem_dnAccLim>"
  BS/23 -> ToWs_Req_Bus_Sig23/1  "<testSig_ExtDem_dnDeclLim>"
  BS/24 -> ToWs_Req_Bus_Sig24/1  "<testSig_ExtDem_facFdbk>"
  BS/25 -> ToWs_Req_Bus_Sig25/1  "<testSig_ExtDem_facFdbkTrqLosHi>"
  BS/26 -> ToWs_Req_Bus_Sig26/1  "<testSig_ExtDem_facFdbkTrqLosLo>"
  BS/27 -> ToWs_Req_Bus_Sig27/1  "<testSig_ExtDem_InrtVehCurr>"
  BS/28 -> ToWs_Req_Bus_Sig28/1  "<testSig_ExtDem_tiFltTrqLosEstCurr>"
  BS/29 -> ToWs_Req_Bus_Sig29/1  "<testSig_ExtDem_KpCorFac_mp>"
  BS/30 -> ToWs_Req_Bus_Sig30/1  "<testSig_ExtDem_KiCorFac_mp>"
  BS/31 -> ToWs_Req_Bus_Sig31/1  "<testSig_ExtDem_Cfg_mp>"
  BS/32 -> ToWs_Req_Bus_Sig32/1  "<testSig_EISGov_st6>"
  BS/33 -> ToWs_Req_Bus_Sig33/1  "<testSig_ExtDem_KpCurrHi_mp>"
  BS/34 -> ToWs_Req_Bus_Sig34/1  "<testSig_ExtDem_KpCurrLo_mp>"
  BS/35 -> ToWs_Req_Bus_Sig35/1  "<testSig_ExtDem_KpNegCurrHi_mp>"
  BS/36 -> ToWs_Req_Bus_Sig36/1  "<testSig_ExtDem_KpNegCurrLo_mp>"
  BS/37 -> ToWs_Req_Bus_Sig37/1  "<testSig_ExtDem_KpPosCurrHi_mp>"
  BS/38 -> ToWs_Req_Bus_Sig38/1  "<testSig_ExtDem_KpPosCurrLo_mp>"
  BS/39 -> ToWs_Req_Bus_Sig39/1  "<testSig_ExtDem_PWinPosHi>"
  BS/40 -> ToWs_Req_Bus_Sig40/1  "<testSig_ExtDem_PWinPosLo>"
  BS/41 -> ToWs_Req_Bus_Sig41/1  "<testSig_ExtDem_PWinNegHi>"
  BS/42 -> ToWs_Req_Bus_Sig42/1  "<testSig_ExtDem_PWinNegLo>"
  BS/43 -> ToWs_Req_Bus_Sig43/1  "<testSig_ExtDem_KiCurrHi_mp>"
  BS/44 -> ToWs_Req_Bus_Sig44/1  "<testSig_ExtDem_KiCurrLo_mp>"
  BS/45 -> ToWs_Req_Bus_Sig45/1  "<testSig_ExtDem_KiNegCurrHi_mp>"
  BS/46 -> ToWs_Req_Bus_Sig46/1  "<testSig_ExtDem_KiNegCurrLo_mp>"
  BS/47 -> ToWs_Req_Bus_Sig47/1  "<testSig_ExtDem_KiPosCurrHi_mp>"
  BS/48 -> ToWs_Req_Bus_Sig48/1  "<testSig_ExtDem_KiPosCurrLo_mp>"
  BS/49 -> ToWs_Req_Bus_Sig49/1  "<testSig_ExtDem_IWinPosHi>"
  BS/50 -> ToWs_Req_Bus_Sig50/1  "<testSig_ExtDem_IWinPosLo>"
  BS/51 -> ToWs_Req_Bus_Sig51/1  "<testSig_ExtDem_IWinNegHi>"
  BS/52 -> ToWs_Req_Bus_Sig52/1  "<testSig_ExtDem_IWinNegLo>"
  BS/53 -> ToWs_Req_Bus_Sig53/1  "<testSig_ExtDem_trqReq>"
  sig_Result_Bus/1 -> BS_Result/1, specifyOutputs/2(sig_Result_Bus)
  BS_Result/1 -> ToWs_Result_Bus_Sig1/1  "<ExtDem_dnAccLim>"
  BS_Result/2 -> ToWs_Result_Bus_Sig2/1  "<ExtDem_dnDeclLim>"
  BS_Result/3 -> ToWs_Result_Bus_Sig3/1  "<ExtDem_facFdbk>"
  BS_Result/4 -> ToWs_Result_Bus_Sig4/1  "<ExtDem_facFdbkTrqLosHi>"
  BS_Result/5 -> ToWs_Result_Bus_Sig5/1  "<ExtDem_facFdbkTrqLosLo>"
  BS_Result/6 -> ToWs_Result_Bus_Sig6/1  "<ExtDem_InrtVehCurr>"
  BS_Result/7 -> ToWs_Result_Bus_Sig7/1  "<ExtDem_tiFltTrqLosEstCurr>"
  BS_Result/8 -> ToWs_Result_Bus_Sig8/1  "<ExtDem_KpCorFac_mp>"
  BS_Result/9 -> ToWs_Result_Bus_Sig9/1  "<ExtDem_KiCorFac_mp>"
  BS_Result/10 -> ToWs_Result_Bus_Sig10/1  "<ExtDem_Cfg_mp>"
  BS_Result/11 -> ToWs_Result_Bus_Sig11/1  "<EISGov_st6>"
  BS_Result/12 -> ToWs_Result_Bus_Sig12/1  "<ExtDem_KpCurrHi_mp>"
  BS_Result/13 -> ToWs_Result_Bus_Sig13/1  "<ExtDem_KpCurrLo_mp>"
  BS_Result/14 -> ToWs_Result_Bus_Sig14/1  "<ExtDem_KpNegCurrHi_mp>"
  BS_Result/15 -> ToWs_Result_Bus_Sig15/1  "<ExtDem_KpNegCurrLo_mp>"
  BS_Result/16 -> ToWs_Result_Bus_Sig16/1  "<ExtDem_KpPosCurrHi_mp>"
  BS_Result/17 -> ToWs_Result_Bus_Sig17/1  "<ExtDem_KpPosCurrLo_mp>"
  BS_Result/18 -> ToWs_Result_Bus_Sig18/1  "<ExtDem_PWinPosHi>"
  BS_Result/19 -> ToWs_Result_Bus_Sig19/1  "<ExtDem_PWinPosLo>"
  BS_Result/20 -> ToWs_Result_Bus_Sig20/1  "<ExtDem_PWinNegHi>"
  BS_Result/21 -> ToWs_Result_Bus_Sig21/1  "<ExtDem_PWinNegLo>"
  BS_Result/22 -> ToWs_Result_Bus_Sig22/1  "<ExtDem_KiCurrHi_mp>"
  BS_Result/23 -> ToWs_Result_Bus_Sig23/1  "<ExtDem_KiCurrLo_mp>"
  BS_Result/24 -> ToWs_Result_Bus_Sig24/1  "<ExtDem_KiNegCurrHi_mp>"
  BS_Result/25 -> ToWs_Result_Bus_Sig25/1  "<ExtDem_KiNegCurrLo_mp>"
  BS_Result/26 -> ToWs_Result_Bus_Sig26/1  "<ExtDem_KiPosCurrHi_mp>"
  BS_Result/27 -> ToWs_Result_Bus_Sig27/1  "<ExtDem_KiPosCurrLo_mp>"
  BS_Result/28 -> ToWs_Result_Bus_Sig28/1  "<ExtDem_IWinPosHi>"
  BS_Result/29 -> ToWs_Result_Bus_Sig29/1  "<ExtDem_IWinPosLo>"
  BS_Result/30 -> ToWs_Result_Bus_Sig30/1  "<ExtDem_IWinNegHi>"
  BS_Result/31 -> ToWs_Result_Bus_Sig31/1  "<ExtDem_IWinNegLo>"
  BS_Result/32 -> ToWs_Result_Bus_Sig32/1  "<ExtDem_trqReq>"
  specifyOutputs/1(result) -> result/1

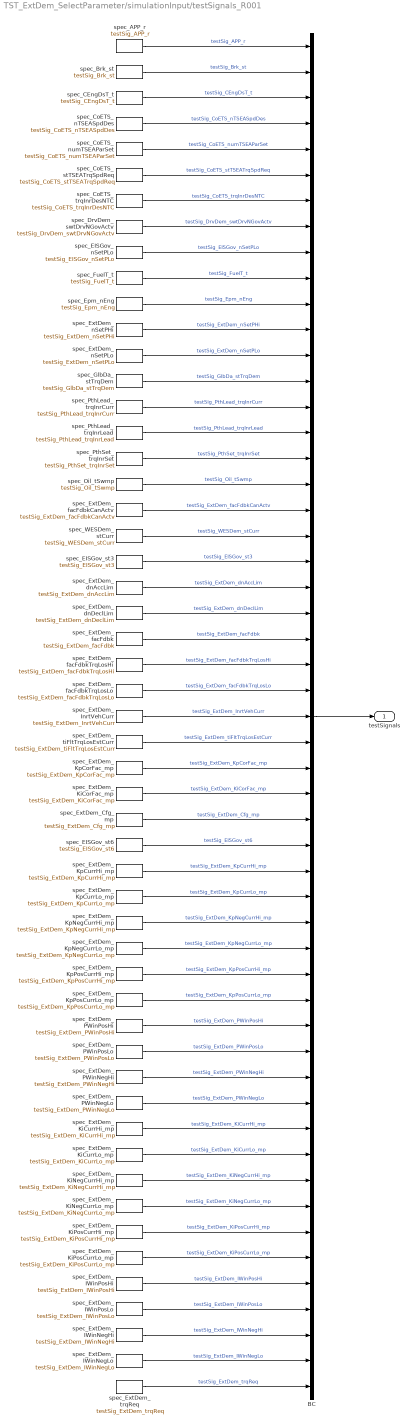
== system TST_ExtDem_SelectParameter/simulationInput/testSignals_R001 ==
  BC : BusCreator  Inputs=53
  spec_APP_r : FromWorkspace  VariableName=testSig_APP_r  Interpolate=off  OutputAfterFinalValue=Holding final value
  spec_Brk_st : FromWorkspace  VariableName=testSig_Brk_st  Interpolate=off  OutputAfterFinalValue=Holding final value
  spec_CEngDsT_t : FromWorkspace  VariableName=testSig_CEngDsT_t  Interpolate=off  OutputAfterFinalValue=Holding final value
  spec_CoETS_nTSEASpdDes : FromWorkspace  VariableName=testSig_CoETS_nTSEASpdDes  Interpolate=off  OutputAfterFinalValue=Holding final value
  spec_CoETS_numTSEAParSet : FromWorkspace  VariableName=testSig_CoETS_numTSEAParSet  Interpolate=off  OutputAfterFinalValue=Holding final value
  spec_CoETS_stTSEATrqSpdReq : FromWorkspace  VariableName=testSig_CoETS_stTSEATrqSpdReq  Interpolate=off  OutputAfterFinalValue=Holding final value
  spec_CoETS_trqInrDesNTC : FromWorkspace  VariableName=testSig_CoETS_trqInrDesNTC  Interpolate=off  OutputAfterFinalValue=Holding final value
  spec_DrvDem_swtDrvNGovActv : FromWorkspace  VariableName=testSig_DrvDem_swtDrvNGovActv  Interpolate=off  OutputAfterFinalValue=Holding final value
  spec_EISGov_nSetPLo : FromWorkspace  VariableName=testSig_EISGov_nSetPLo  Interpolate=off  OutputAfterFinalValue=Holding final value
  spec_EISGov_st3 : FromWorkspace  VariableName=testSig_EISGov_st3  Interpolate=off  OutputAfterFinalValue=Holding final value
  spec_EISGov_st6 : FromWorkspace  VariableName=testSig_EISGov_st6  Interpolate=off  OutputAfterFinalValue=Holding final value
  spec_Epm_nEng : FromWorkspace  VariableName=testSig_Epm_nEng  Interpolate=off  OutputAfterFinalValue=Holding final value
  spec_ExtDem_Cfg_mp : FromWorkspace  VariableName=testSig_ExtDem_Cfg_mp  Interpolate=off  OutputAfterFinalValue=Holding final value
  spec_ExtDem_IWinNegHi : FromWorkspace  VariableName=testSig_ExtDem_IWinNegHi  Interpolate=off  OutputAfterFinalValue=Holding final value
  spec_ExtDem_IWinNegLo : FromWorkspace  VariableName=testSig_ExtDem_IWinNegLo  Interpolate=off  OutputAfterFinalValue=Holding final value
  spec_ExtDem_IWinPosHi : FromWorkspace  VariableName=testSig_ExtDem_IWinPosHi  Interpolate=off  OutputAfterFinalValue=Holding final value
  spec_ExtDem_IWinPosLo : FromWorkspace  VariableName=testSig_ExtDem_IWinPosLo  Interpolate=off  OutputAfterFinalValue=Holding final value
  spec_ExtDem_InrtVehCurr : FromWorkspace  VariableName=testSig_ExtDem_InrtVehCurr  Interpolate=off  OutputAfterFinalValue=Holding final value
  spec_ExtDem_KiCorFac_mp : FromWorkspace  VariableName=testSig_ExtDem_KiCorFac_mp  Interpolate=off  OutputAfterFinalValue=Holding final value
  spec_ExtDem_KiCurrHi_mp : FromWorkspace  VariableName=testSig_ExtDem_KiCurrHi_mp  Interpolate=off  OutputAfterFinalValue=Holding final value
  spec_ExtDem_KiCurrLo_mp : FromWorkspace  VariableName=testSig_ExtDem_KiCurrLo_mp  Interpolate=off  OutputAfterFinalValue=Holding final value
  spec_ExtDem_KiNegCurrHi_mp : FromWorkspace  VariableName=testSig_ExtDem_KiNegCurrHi_mp  Interpolate=off  OutputAfterFinalValue=Holding final value
  spec_ExtDem_KiNegCurrLo_mp : FromWorkspace  VariableName=testSig_ExtDem_KiNegCurrLo_mp  Interpolate=off  OutputAfterFinalValue=Holding final value
  spec_ExtDem_KiPosCurrHi_mp : FromWorkspace  VariableName=testSig_ExtDem_KiPosCurrHi_mp  Interpolate=off  OutputAfterFinalValue=Holding final value
  spec_ExtDem_KiPosCurrLo_mp : FromWorkspace  VariableName=testSig_ExtDem_KiPosCurrLo_mp  Interpolate=off  OutputAfterFinalValue=Holding final value
  spec_ExtDem_KpCorFac_mp : FromWorkspace  VariableName=testSig_ExtDem_KpCorFac_mp  Interpolate=off  OutputAfterFinalValue=Holding final value
  spec_ExtDem_KpCurrHi_mp : FromWorkspace  VariableName=testSig_ExtDem_KpCurrHi_mp  Interpolate=off  OutputAfterFinalValue=Holding final value
  spec_ExtDem_KpCurrLo_mp : FromWorkspace  VariableName=testSig_ExtDem_KpCurrLo_mp  Interpolate=off  OutputAfterFinalValue=Holding final value
  spec_ExtDem_KpNegCurrHi_mp : FromWorkspace  VariableName=testSig_ExtDem_KpNegCurrHi_mp  Interpolate=off  OutputAfterFinalValue=Holding final value
  spec_ExtDem_KpNegCurrLo_mp : FromWorkspace  VariableName=testSig_ExtDem_KpNegCurrLo_mp  Interpolate=off  OutputAfterFinalValue=Holding final value
  spec_ExtDem_KpPosCurrHi_mp : FromWorkspace  VariableName=testSig_ExtDem_KpPosCurrHi_mp  Interpolate=off  OutputAfterFinalValue=Holding final value
  spec_ExtDem_KpPosCurrLo_mp : FromWorkspace  VariableName=testSig_ExtDem_KpPosCurrLo_mp  Interpolate=off  OutputAfterFinalValue=Holding final value
  spec_ExtDem_PWinNegHi : FromWorkspace  VariableName=testSig_ExtDem_PWinNegHi  Interpolate=off  OutputAfterFinalValue=Holding final value
  spec_ExtDem_PWinNegLo : FromWorkspace  VariableName=testSig_ExtDem_PWinNegLo  Interpolate=off  OutputAfterFinalValue=Holding final value
  spec_ExtDem_PWinPosHi : FromWorkspace  VariableName=testSig_ExtDem_PWinPosHi  Interpolate=off  OutputAfterFinalValue=Holding final value
  spec_ExtDem_PWinPosLo : FromWorkspace  VariableName=testSig_ExtDem_PWinPosLo  Interpolate=off  OutputAfterFinalValue=Holding final value
  spec_ExtDem_dnAccLim : FromWorkspace  VariableName=testSig_ExtDem_dnAccLim  Interpolate=off  OutputAfterFinalValue=Holding final value
  spec_ExtDem_dnDeclLim : FromWorkspace  VariableName=testSig_ExtDem_dnDeclLim  Interpolate=off  OutputAfterFinalValue=Holding final value
  spec_ExtDem_facFdbk : FromWorkspace  VariableName=testSig_ExtDem_facFdbk  Interpolate=off  OutputAfterFinalValue=Holding final value
  spec_ExtDem_facFdbkCanActv : FromWorkspace  VariableName=testSig_ExtDem_facFdbkCanActv  Interpolate=off  OutputAfterFinalValue=Holding final value
  spec_ExtDem_facFdbkTrqLosHi : FromWorkspace  VariableName=testSig_ExtDem_facFdbkTrqLosHi  Interpolate=off  OutputAfterFinalValue=Holding final value
  spec_ExtDem_facFdbkTrqLosLo : FromWorkspace  VariableName=testSig_ExtDem_facFdbkTrqLosLo  Interpolate=off  OutputAfterFinalValue=Holding final value
  spec_ExtDem_nSetPHi : FromWorkspace  VariableName=testSig_ExtDem_nSetPHi  Interpolate=off  OutputAfterFinalValue=Holding final value
  spec_ExtDem_nSetPLo : FromWorkspace  VariableName=testSig_ExtDem_nSetPLo  Interpolate=off  OutputAfterFinalValue=Holding final value
  spec_ExtDem_tiFltTrqLosEstCurr : FromWorkspace  VariableName=testSig_ExtDem_tiFltTrqLosEstCurr  Interpolate=off  OutputAfterFinalValue=Holding final value
  spec_ExtDem_trqReq : FromWorkspace  VariableName=testSig_ExtDem_trqReq  Interpolate=off  OutputAfterFinalValue=Holding final value
  spec_FuelT_t : FromWorkspace  VariableName=testSig_FuelT_t  Interpolate=off  OutputAfterFinalValue=Holding final value
  spec_GlbDa_stTrqDem : FromWorkspace  VariableName=testSig_GlbDa_stTrqDem  Interpolate=off  OutputAfterFinalValue=Holding final value
  spec_Oil_tSwmp : FromWorkspace  VariableName=testSig_Oil_tSwmp  Interpolate=off  OutputAfterFinalValue=Holding final value
  spec_PthLead_trqInrCurr : FromWorkspace  VariableName=testSig_PthLead_trqInrCurr  Interpolate=off  OutputAfterFinalValue=Holding final value
  spec_PthLead_trqInrLead : FromWorkspace  VariableName=testSig_PthLead_trqInrLead  Interpolate=off  OutputAfterFinalValue=Holding final value
  spec_PthSet_trqInrSet : FromWorkspace  VariableName=testSig_PthSet_trqInrSet  Interpolate=off  OutputAfterFinalValue=Holding final value
  spec_WESDem_stCurr : FromWorkspace  VariableName=testSig_WESDem_stCurr  Interpolate=off  OutputAfterFinalValue=Holding final value
  testSignals : Outport
  wires:
  BC/1 -> testSignals/1
  spec_APP_r/1 -> BC/1  "testSig_APP_r"
  spec_Brk_st/1 -> BC/2  "testSig_Brk_st"
  spec_CEngDsT_t/1 -> BC/3  "testSig_CEngDsT_t"
  spec_CoETS_nTSEASpdDes/1 -> BC/4  "testSig_CoETS_nTSEASpdDes"
  spec_CoETS_numTSEAParSet/1 -> BC/5  "testSig_CoETS_numTSEAParSet"
  spec_CoETS_stTSEATrqSpdReq/1 -> BC/6  "testSig_CoETS_stTSEATrqSpdReq"
  spec_CoETS_trqInrDesNTC/1 -> BC/7  "testSig_CoETS_trqInrDesNTC"
  spec_DrvDem_swtDrvNGovActv/1 -> BC/8  "testSig_DrvDem_swtDrvNGovActv"
  spec_EISGov_nSetPLo/1 -> BC/9  "testSig_EISGov_nSetPLo"
  spec_FuelT_t/1 -> BC/10  "testSig_FuelT_t"
  spec_Epm_nEng/1 -> BC/11  "testSig_Epm_nEng"
  spec_ExtDem_nSetPHi/1 -> BC/12  "testSig_ExtDem_nSetPHi"
  spec_ExtDem_nSetPLo/1 -> BC/13  "testSig_ExtDem_nSetPLo"
  spec_GlbDa_stTrqDem/1 -> BC/14  "testSig_GlbDa_stTrqDem"
  spec_PthLead_trqInrCurr/1 -> BC/15  "testSig_PthLead_trqInrCurr"
  spec_PthLead_trqInrLead/1 -> BC/16  "testSig_PthLead_trqInrLead"
  spec_PthSet_trqInrSet/1 -> BC/17  "testSig_PthSet_trqInrSet"
  spec_Oil_tSwmp/1 -> BC/18  "testSig_Oil_tSwmp"
  spec_ExtDem_facFdbkCanActv/1 -> BC/19  "testSig_ExtDem_facFdbkCanActv"
  spec_WESDem_stCurr/1 -> BC/20  "testSig_WESDem_stCurr"
  spec_EISGov_st3/1 -> BC/21  "testSig_EISGov_st3"
  spec_ExtDem_dnAccLim/1 -> BC/22  "testSig_ExtDem_dnAccLim"
  spec_ExtDem_dnDeclLim/1 -> BC/23  "testSig_ExtDem_dnDeclLim"
  spec_ExtDem_facFdbk/1 -> BC/24  "testSig_ExtDem_facFdbk"
  spec_ExtDem_facFdbkTrqLosHi/1 -> BC/25  "testSig_ExtDem_facFdbkTrqLosHi"
  spec_ExtDem_facFdbkTrqLosLo/1 -> BC/26  "testSig_ExtDem_facFdbkTrqLosLo"
  spec_ExtDem_InrtVehCurr/1 -> BC/27  "testSig_ExtDem_InrtVehCurr"
  spec_ExtDem_tiFltTrqLosEstCurr/1 -> BC/28  "testSig_ExtDem_tiFltTrqLosEstCurr"
  spec_ExtDem_KpCorFac_mp/1 -> BC/29  "testSig_ExtDem_KpCorFac_mp"
  spec_ExtDem_KiCorFac_mp/1 -> BC/30  "testSig_ExtDem_KiCorFac_mp"
  spec_ExtDem_Cfg_mp/1 -> BC/31  "testSig_ExtDem_Cfg_mp"
  spec_EISGov_st6/1 -> BC/32  "testSig_EISGov_st6"
  spec_ExtDem_KpCurrHi_mp/1 -> BC/33  "testSig_ExtDem_KpCurrHi_mp"
  spec_ExtDem_KpCurrLo_mp/1 -> BC/34  "testSig_ExtDem_KpCurrLo_mp"
  spec_ExtDem_KpNegCurrHi_mp/1 -> BC/35  "testSig_ExtDem_KpNegCurrHi_mp"
  spec_ExtDem_KpNegCurrLo_mp/1 -> BC/36  "testSig_ExtDem_KpNegCurrLo_mp"
  spec_ExtDem_KpPosCurrHi_mp/1 -> BC/37  "testSig_ExtDem_KpPosCurrHi_mp"
  spec_ExtDem_KpPosCurrLo_mp/1 -> BC/38  "testSig_ExtDem_KpPosCurrLo_mp"
  spec_ExtDem_PWinPosHi/1 -> BC/39  "testSig_ExtDem_PWinPosHi"
  spec_ExtDem_PWinPosLo/1 -> BC/40  "testSig_ExtDem_PWinPosLo"
  spec_ExtDem_PWinNegHi/1 -> BC/41  "testSig_ExtDem_PWinNegHi"
  spec_ExtDem_PWinNegLo/1 -> BC/42  "testSig_ExtDem_PWinNegLo"
  spec_ExtDem_KiCurrHi_mp/1 -> BC/43  "testSig_ExtDem_KiCurrHi_mp"
  spec_ExtDem_KiCurrLo_mp/1 -> BC/44  "testSig_ExtDem_KiCurrLo_mp"
  spec_ExtDem_KiNegCurrHi_mp/1 -> BC/45  "testSig_ExtDem_KiNegCurrHi_mp"
  spec_ExtDem_KiNegCurrLo_mp/1 -> BC/46  "testSig_ExtDem_KiNegCurrLo_mp"
  spec_ExtDem_KiPosCurrHi_mp/1 -> BC/47  "testSig_ExtDem_KiPosCurrHi_mp"
  spec_ExtDem_KiPosCurrLo_mp/1 -> BC/48  "testSig_ExtDem_KiPosCurrLo_mp"
  spec_ExtDem_IWinPosHi/1 -> BC/49  "testSig_ExtDem_IWinPosHi"
  spec_ExtDem_IWinPosLo/1 -> BC/50  "testSig_ExtDem_IWinPosLo"
  spec_ExtDem_IWinNegHi/1 -> BC/51  "testSig_ExtDem_IWinNegHi"
  spec_ExtDem_IWinNegLo/1 -> BC/52  "testSig_ExtDem_IWinNegLo"
  spec_ExtDem_trqReq/1 -> BC/53  "testSig_ExtDem_trqReq"
